simulink model "MGTestSystem_4bus"  (R2021b)
settings: Solver=VariableStepAuto  StartTime=0.0  StopTime=4  RelTol=1e-3
PreLoadFcn:
  | addpath Icons
  | addpath Util
InitFcn:
  | clc
  | %clear all
  | 
  | nDER = 4;
  | xssum = zeros(nDER*2,1);
  | save XSSUM xssum
  | 
  | Ts_Control=1e-4;       % local control time step
  | Ts_Simulation=5e-5;   %simulation time step
  | Ts_Power=5e-5;   % measurement time step
  | Tdisc=0.8;     % time setting for disconnecting from the main grid
  | 
  | Iref = 0.3;  % in p.u.
  | Iqref = 0;  % in p.u.
  | 
  | Ts_secondary =3e-2;   %  secondary control time step
  | %Ts_PMU = 1/60;
  | 
  | ft2km=3.0480e-04;
  | 
  | KPdroop=3.4e-4;
  | KQdroop=1e-3/1;
  | KPdroop2=4.5e-4;
  | KQdroop2=1.5e-3/1;
  | 
  | %KWinvdroop = 20.0;
  | %KVinvdroop = 16.7;
  | %KWinvdroop = 0.05;
  | %KVinvdroop = 0.08;
  | 
  | KWinvdroop = 1/(2*pi*KPdroop);
  | KVinvdroop = 1/(2*pi*KQdroop)
  | KWinvdroop2 = 1/(2*pi*KPdroop2);
  | KVinvdroop2 = 1/(2*pi*KQdroop2)
  | %KVinvdroop = 1/(KQdroop);
  | %KVinvdroop2 = 1/(KQdroop2);
  | %KWinvdroop = 1/(KPdroop);
  | %KWinvdroop2 = 1/(KPdroop2);
  | 
  | droopv1=1/KVinvdroop
  | droopv2=1/KVinvdroop2
  | 
  | 
  | 
  | 
  | wfilter = 35;
  | Rv=0.0;
  | Lv=0e-3;
  | 
  | div=1;
  | 
  | 
  | Kpac=0.1/1;
  | Kiac=420/1;
  | Kpaci=15/div;
  | Kiaci=2e3/div;
  | Kpac2=0.05/1;
  | Kiac2=390/1;
  | Kpaci2=15/div;
  | Kiaci2=1.6e3/div;
  | ... (+47 lines)
undefined symbols (not defined in the file or in its folder): D1, Delta, Ion, Lithium
libraries: spsStairGeneratorLib x24, spsThreePhaseSeriesRLCBranchLib x24, powerlib_extras x23, spsSeriesRLCBranchLib x20, spsThreePhaseVIMeasurementLib x18, slpidlib x18, spsThreePhaseBreakerLib x15, spsRMSLib x10, spsThreePhaseSeriesRLCLoadLib x8, spsVoltageMeasurementLib x8, spsPMUPLLBasedPositiveSequenceLib x6, spsPowerLib x5
(part 3 of 7)

== system MGTestSystem_4bus/Bus_6/PLL ==
  Vabc_LN_pu : Inport
  2pi60'1 : Constant  Value=2*pi*60
  2pi60'2 : Constant  Value=2*pi*60
  2pi60'3 : Constant  Value=2*pi*60
  Constant : Constant  Value=90
  Demux : Demux  Outputs=3
  Gain1 : Gain  Gain=180/pi  SaturateOnIntegerOverflow=on  OutDataTypeStr=Inherit: Same as input  ParamDataTypeStr=Inherit: Same as input
  Gain2 : Gain  Gain=180/pi  SaturateOnIntegerOverflow=on  OutDataTypeStr=Inherit: Same as input  ParamDataTypeStr=Inherit: Same as input
  Gain3 : Gain  Gain=180/pi  SaturateOnIntegerOverflow=on  OutDataTypeStr=Inherit: Same as input  ParamDataTypeStr=Inherit: Same as input
  Mux : Mux  Inputs=3
  Pll1 : Subsystem
  Pll2 : Subsystem
  Pll3 : Subsystem
  Sum : Sum  Inputs=|++
  delta_abc : Outport  VectorParamsAs1DForOutWhenUnconnected=off
  wires:
  Vabc_LN_pu/1 -> Demux/1
  Demux/1 -> Pll3/1(señal)
  2pi60'3/1 -> Pll3/2(w)
  Pll3/1(f cos (rad)) -> Gain1/1
  Demux/2 -> Pll1/1(señal)
  2pi60'1/1 -> Pll1/2(w)
  Gain2/1 -> Mux/2
  Demux/3 -> Pll2/1(señal)
  2pi60'2/1 -> Pll2/2(w)
  Pll2/1(f cos (rad)) -> Gain3/1
  Gain3/1 -> Mux/3
  Pll1/1(f cos (rad)) -> Gain2/1
  Mux/1 -> Sum/1
  Gain1/1 -> Mux/1
  Constant/1 -> Sum/2
  Sum/1 -> delta_abc/1

== system MGTestSystem_4bus/Bus_6/Power Factor Block1 ==
  Vabc : Inport
  Iabc : Inport  Port=2
  Complex to Magnitude-Angle : ComplexToMagnitudeAngle
  Mux : Mux  Inputs=2
  Mux1 : Mux  Inputs=2
  Power : spsPowerLib/Power  Freq=Freq  Vinit=Vinit  Iinit=Iinit  Ts=Ts
      settings: SourceProductBaseCode=PS
  RMS3 : spsRMSLib/RMS  TrueRMS=on  Freq=60  RMSInit=0  Ts=Ts_Simulation
  RMS4 : spsRMSLib/RMS  TrueRMS=on  Freq=60  RMSInit=0  Ts=Ts_Simulation
  Real-Imag to Complex : RealImagToComplex
  Terminator : Terminator
  compara : Gain  SaturateOnIntegerOverflow=on  OutDataTypeStr=Inherit: Same as input  ParamDataTypeStr=Inherit: Same as input
  cos(theta) : Trigonometry  Operator=cos
  to Kw : Gain  Gain=1/1000
  to Kw1 : Gain  Gain=1/1000
  Pabc : Outport  VectorParamsAs1DForOutWhenUnconnected=off
  Qabc : Outport  Port=2  VectorParamsAs1DForOutWhenUnconnected=off
  Vabc y Vabc (rms) : Outport  Port=3  VectorParamsAs1DForOutWhenUnconnected=off
  Iabc y Iabc (rms) : Outport  Port=4  VectorParamsAs1DForOutWhenUnconnected=off
  "PFabc " : Outport  Port=5  VectorParamsAs1DForOutWhenUnconnected=off
  tag scope: P_abc_Bus0=global, Q_abc_Bus0=global
  wires:
  Complex to Magnitude-Angle/2 -> cos(theta)/1
  Real-Imag to Complex/1 -> Complex to Magnitude-Angle/1
  cos(theta)/1 -> "PFabc "/1
  Complex to Magnitude-Angle/1 -> Terminator/1
  Iabc/1 -> RMS4/1, compara/1, Power/2
  RMS4/1 -> Mux1/2
  Mux1/1 -> Iabc y Iabc (rms)/1
  Mux/1 -> Vabc y Vabc (rms)/1
  Vabc/1 -> Power/1, Mux/2, RMS3/1
  compara/1 -> Mux1/1
  RMS3/1 -> Mux/1
  Power/1 -> to Kw1/1, Pabc/1, Real-Imag to Complex/1
  Power/2 -> Qabc/1, Real-Imag to Complex/2, to Kw/1
  to Kw/1 -> [Q_abc_Bus0]
  to Kw1/1 -> [P_abc_Bus0]

== system MGTestSystem_4bus/DATA  ADQUISITION/Delta_abc ==
  From10 : From  Commented=on  GotoTag=delta_abc_Bus8  TagVisibility=global
  From12 : From  Commented=on  GotoTag=delta_abc_Bus9  TagVisibility=global
  From13 : From  Commented=on  GotoTag=delta_abc_Bus10  TagVisibility=global
  From14 : From  Commented=on  GotoTag=delta_abc_Bus5  TagVisibility=global
  From15 : From  Commented=on  GotoTag=delta_abc_Bus11  TagVisibility=global
  From16 : From  Commented=on  GotoTag=delta_abc_Bus12  TagVisibility=global
  From17 : From  Commented=on  GotoTag=delta_abc_Bus13  TagVisibility=global
  From18 : From  Commented=on  GotoTag=delta_abc_Bus4L  TagVisibility=global
  From20 : From  Commented=on  GotoTag=delta_abc_Bus6  TagVisibility=global
  From22 : From  Commented=on  GotoTag=delta_abc_Bus4L  TagVisibility=global
  From23 : From  Commented=on  GotoTag=delta_abc_Bus7  TagVisibility=global
  From24 : From  Commented=on  GotoTag=delta_abc_Bus5L  TagVisibility=global
  From26 : From  Commented=on  GotoTag=delta_abc_Bus8  TagVisibility=global
  From29 : From  Commented=on  GotoTag=delta_abc_Bus9  TagVisibility=global
  From3 : From  Commented=on  GotoTag=delta_abc_Bus5  TagVisibility=global
  From32 : From  Commented=on  GotoTag=delta_abc_Bus10  TagVisibility=global
  From35 : From  Commented=on  GotoTag=delta_abc_Bus11  TagVisibility=global
  From38 : From  Commented=on  GotoTag=delta_abc_Bus12  TagVisibility=global
  From4 : From  Commented=on  GotoTag=delta_abc_Bus13  TagVisibility=global
  From41 : From  Commented=on  GotoTag=delta_abc_Bus4L  TagVisibility=global
  From7 : From  Commented=on  GotoTag=delta_abc_Bus6  TagVisibility=global
  From9 : From  Commented=on  GotoTag=delta_abc_Bus7  TagVisibility=global
  Mux3 : Mux  Inputs=15
  Scope : Scope  Commented=on  NumInputPorts=15
  f3 : ToWorkspace  Commented=on  VariableName=ang_abc  SaveFormat=Timeseries  SampleTime=-1
  wires:
  From32/1 -> Mux3/10
  [delta_abc_Bus4] -> Mux3/4
  From23/1 -> Mux3/7
  From26/1 -> Mux3/8
  From35/1 -> Mux3/11
  From14/1 -> Mux3/5
  From29/1 -> Mux3/9
  [delta_abc_Bus2] -> Mux3/2
  [delta_abc_Bus1] -> Mux3/1
  From38/1 -> Mux3/12
  From41/1 -> Mux3/14
  Mux3/1 -> f3/1
  From20/1 -> Mux3/6
  From17/1 -> Mux3/13
  [delta_abc_Bus3] -> Mux3/3
  [delta_abc_Bus3] -> Scope/3
  From4/1 -> Scope/13
  From7/1 -> Scope/6
  From13/1 -> Scope/10
  [delta_abc_Bus2] -> Scope/2
  [delta_abc_Bus1] -> Scope/1
  From3/1 -> Scope/5
  From16/1 -> Scope/12
  From15/1 -> Scope/11
  From10/1 -> Scope/8
  From18/1 -> Scope/14
  From12/1 -> Scope/9
  From9/1 -> Scope/7
  [delta_abc_Bus4] -> Scope/4
  From22/1 -> Scope/15
  From24/1 -> Mux3/15

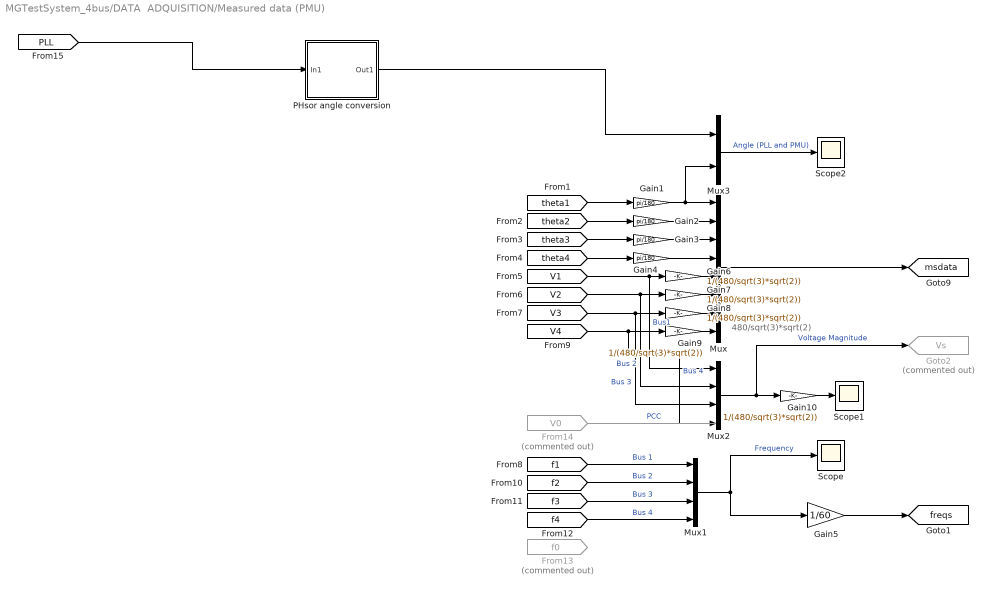
== system MGTestSystem_4bus/DATA  ADQUISITION/Measured data (PMU) ==
  note: 480/sqrt(3)*sqrt(2)
  From13 : From  Commented=on  GotoTag=f0  TagVisibility=global
  From14 : From  Commented=on  GotoTag=V0  TagVisibility=global
  Gain{1..4} (4 alike) : Gain  Gain=pi/180
  Gain{6..10} (5 alike) : Gain  Gain=1/(480/sqrt(3)*sqrt(2))
  Gain5 : Gain  Gain=1/60
  Goto2 : Goto  Commented=on  GotoTag=Vs  TagVisibility=global
  Mux : Mux  Inputs=8
  Mux1 : Mux
  Mux2 : Mux
  Mux3 : Mux  Inputs=2
  PHsor angle conversion : Subsystem
  Scope : Scope
  Scope1 : Scope
  Scope2 : Scope
  tag scope: freqs=global, msdata=global
  wires:
  [theta1] -> Gain1/1
  Mux/1 -> [msdata]
  [theta2] -> Gain2/1
  [V2] -> Mux2/2, Gain7/1  "Bus 2"
  [V3] -> Mux2/3, Gain8/1  "Bus 3"
  [V4] -> Mux2/4, Gain9/1  "Bus 4"
  [theta3] -> Gain3/1
  [theta4] -> Gain4/1
  [f1] -> Mux1/1  "Bus 1"
  [f2] -> Mux1/2  "Bus 2"
  [f3] -> Mux1/3  "Bus 3"
  [f4] -> Mux1/4  "Bus 4"
  Mux1/1 -> Scope/1, Gain5/1  "Frequency"
  [V1] -> Mux2/1, Gain6/1  "Bus1"
  Mux2/1 -> Goto2/1, Gain10/1  "Voltage Magnitude"
  Gain1/1 -> Mux3/2, Mux/1
  Gain2/1 -> Mux/2
  Gain3/1 -> Mux/3
  Gain4/1 -> Mux/4
  Gain5/1 -> [freqs]
  Gain6/1 -> Mux/5
  Gain7/1 -> Mux/6
  Gain8/1 -> Mux/7
  Gain9/1 -> Mux/8
  From14/1 -> ?  "PCC"
  Mux3/1 -> Scope2/1  "Angle (PLL and PMU)"
  [PLL] -> PHsor angle conversion/1(In1)
  PHsor angle conversion/1(Out1) -> Mux3/1
  Gain10/1 -> Scope1/1

== system MGTestSystem_4bus/DATA  ADQUISITION/PF_abc ==
  From11 : From  Commented=on  GotoTag=PFabc_Bus5  TagVisibility=global
  From17 : From  Commented=on  GotoTag=PFabc_Bus6  TagVisibility=global
  From20 : From  Commented=on  GotoTag=PFabc_Bus7  TagVisibility=global
  From23 : From  Commented=on  GotoTag=PFabc_Bus8  TagVisibility=global
  From26 : From  Commented=on  GotoTag=PFabc_Bus9  TagVisibility=global
  From29 : From  Commented=on  GotoTag=PFabc_Bus10  TagVisibility=global
  From32 : From  Commented=on  GotoTag=PFabc_Bus11  TagVisibility=global
  From35 : From  Commented=on  GotoTag=PFabc_Bus12  TagVisibility=global
  From38 : From  Commented=on  GotoTag=PFabc_Bus13  TagVisibility=global
  From41 : From  Commented=on  GotoTag=PFabc_Bus4L  TagVisibility=global
  Mux2 : Mux  Inputs=14
  f3 : ToWorkspace  Commented=on  VariableName=PF_abc  SaveFormat=Timeseries  SampleTime=-1
  wires:
  [PFabc_Bus2] -> Mux2/2
  [PFabc_Bus4] -> Mux2/4
  [PFabc_Bus1] -> Mux2/1
  From17/1 -> Mux2/6
  Mux2/1 -> f3/1
  From11/1 -> Mux2/5
  From41/1 -> Mux2/14
  From23/1 -> Mux2/8
  From26/1 -> Mux2/9
  From20/1 -> Mux2/7
  From32/1 -> Mux2/11
  From38/1 -> Mux2/13
  From29/1 -> Mux2/10
  [PFabc_Bus3] -> Mux2/3
  From35/1 -> Mux2/12

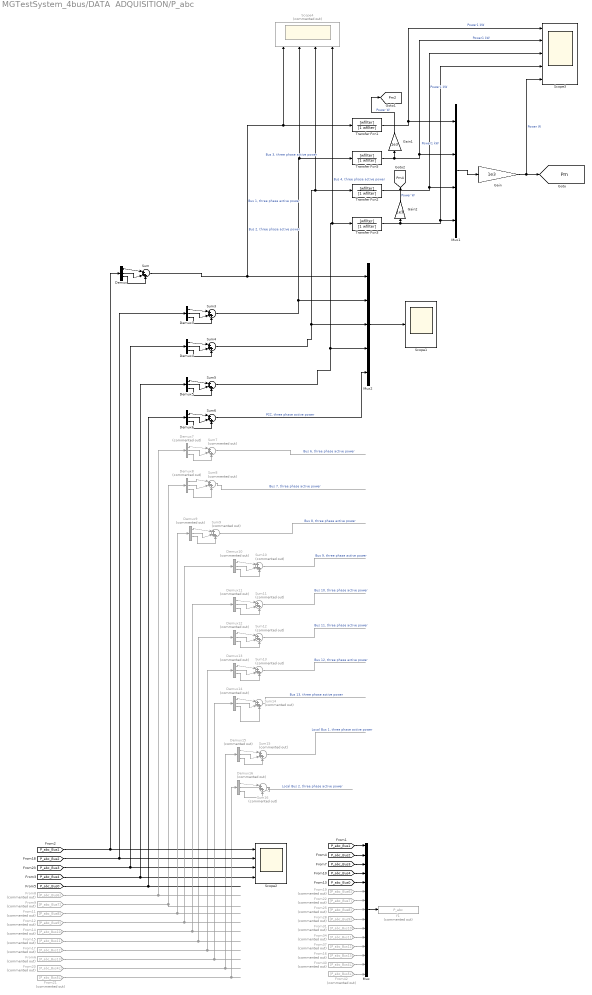
== system MGTestSystem_4bus/DATA  ADQUISITION/P_abc ==
  Demux{,3..6} (5 alike) : Demux  Outputs=3
  Demux{7..16} (10 alike) : Demux  Commented=on  Outputs=3
  From11 : From  Commented=on  GotoTag=P_abc_Bus8  TagVisibility=global
  From12 : From  Commented=on  GotoTag=P_abc_Bus9  TagVisibility=global
  From14 : From  Commented=on  GotoTag=P_abc_Bus10  TagVisibility=global
  From15 : From  Commented=on  GotoTag=P_abc_Bus11  TagVisibility=global
  From16 : From  Commented=on  GotoTag=P_abc_Bus13  TagVisibility=global
  From17 : From  Commented=on  GotoTag=P_abc_Bus12  TagVisibility=global
  From19 : From  Commented=on  GotoTag=P_abc_Bus6  TagVisibility=global
  From20 : From  Commented=on  GotoTag=P_abc_Bus4L  TagVisibility=global
  From21 : From  Commented=on  GotoTag=P_abc_Bus5L  TagVisibility=global
  From22 : From  Commented=on  GotoTag=P_abc_Bus7  TagVisibility=global
  From25 : From  Commented=on  GotoTag=P_abc_Bus8  TagVisibility=global
  From28 : From  Commented=on  GotoTag=P_abc_Bus9  TagVisibility=global
  From31 : From  Commented=on  GotoTag=P_abc_Bus10  TagVisibility=global
  From34 : From  Commented=on  GotoTag=P_abc_Bus11  TagVisibility=global
  From37 : From  Commented=on  GotoTag=P_abc_Bus12  TagVisibility=global
  From40 : From  Commented=on  GotoTag=P_abc_Bus4L  TagVisibility=global
  From42 : From  Commented=on  GotoTag=P_abc_Bus5L  TagVisibility=global
  From6 : From  Commented=on  GotoTag=P_abc_Bus13  TagVisibility=global
  From8 : From  Commented=on  GotoTag=P_abc_Bus6  TagVisibility=global
  From9 : From  Commented=on  GotoTag=P_abc_Bus7  TagVisibility=global
  Gain : Gain  Gain=1e3
  Gain1 : Gain  Gain=1e3
  Gain2 : Gain  Gain=1e3
  Mux : Mux  Inputs=15
  Mux1 : Mux
  Mux2 : Mux  Inputs=5
  Scope1 : Scope
  Scope2 : Scope  NumInputPorts=4
  Scope3 : Scope  NumInputPorts=5
  Scope4 : Scope  Commented=on  NumInputPorts=4
  Sum{,3..6} (5 alike) : Sum  Inputs=|+++
  Sum{7..16} (10 alike) : Sum  Commented=on  Inputs=|+++
  Transfer Fcn{1..3,5} (4 alike) : TransferFcn  Numerator=[wfilter]  Denominator=[1 wfilter]
  f1 : ToWorkspace  Commented=on  VariableName=P_abc  SaveFormat=Timeseries  SampleTime=-1
  tag scope: Pm2=global, Pm4=global, Pm=global
  wires:
  [P_abc_Bus1] -> Mux/1
  [P_abc_Bus3] -> Mux/3
  [P_abc_Bus2] -> Mux/2
  From16/1 -> Mux/13
  Mux/1 -> f1/1
  From37/1 -> Mux/12
  From28/1 -> Mux/9
  From25/1 -> Mux/8
  From31/1 -> Mux/10
  From34/1 -> Mux/11
  From22/1 -> Mux/7
  [P_abc_Bus4] -> Mux/4
  From40/1 -> Mux/14
  [P_abc_Bus0] -> Mux/5
  From42/1 -> Mux/15
  From19/1 -> Mux/6
  [P_abc_Bus4] -> Scope2/4, Demux5/1
  From17/1 -> Demux13/1
  From20/1 -> Demux15/1
  From15/1 -> Demux12/1
  From9/1 -> Demux8/1
  [P_abc_Bus3] -> Scope2/3, Demux4/1
  [P_abc_Bus2] -> Scope2/2, Demux3/1
  From6/1 -> Demux14/1
  From12/1 -> Demux10/1
  [P_abc_Bus0] -> Demux6/1
  From21/1 -> Demux16/1
  From8/1 -> Demux7/1
  [P_abc_Bus1] -> Scope2/1, Demux/1
  Demux/1 -> Sum/1
  Demux/2 -> Sum/2
  Demux/3 -> Sum/3
  Sum/1 -> Mux2/1, Transfer Fcn1/1, Scope4/1  "Bus 1, three phase active power"
  From11/1 -> Demux9/1
  From14/1 -> Demux11/1
  Demux3/3 -> Sum3/3
  Demux3/2 -> Sum3/2
  Sum3/1 -> Mux2/2, Transfer Fcn5/1, Scope4/2  "Bus 2, three phase active power"
  Demux3/1 -> Sum3/1
  Demux4/1 -> Sum4/1
  Sum4/1 -> Mux2/3, Transfer Fcn2/1, Scope4/3  "Bus 3, three phase active power"
  Demux4/2 -> Sum4/2
  Demux4/3 -> Sum4/3
  Demux5/3 -> Sum5/3
  Demux5/2 -> Sum5/2
  Sum5/1 -> Mux2/4, Transfer Fcn3/1, Scope4/4  "Bus 4, three phase active power"
  Demux5/1 -> Sum5/1
  Demux6/1 -> Sum6/1
  Sum6/1 -> Mux2/5  "PCC, three phase active power"
  Demux6/2 -> Sum6/2
  Demux6/3 -> Sum6/3
  Demux7/3 -> Sum7/3
  Demux7/2 -> Sum7/2
  Sum7/1 -> ?  "Bus 6, three phase active power"
  Demux7/1 -> Sum7/1
  Demux8/1 -> Sum8/1
  Sum8/1 -> ?  "Bus 7, three phase active power"
  Demux8/2 -> Sum8/2
  Demux8/3 -> Sum8/3
  Demux13/3 -> Sum13/3
  Sum13/1 -> ?  "Bus 12, three phase active power"
  Demux13/1 -> Sum13/1
  Demux13/2 -> Sum13/2
  Sum11/1 -> ?  "Bus 10, three phase active power"
  Demux11/1 -> Sum11/1
  Demux11/3 -> Sum11/3
  Demux11/2 -> Sum11/2
  Demux12/2 -> Sum12/2
  Sum12/1 -> ?  "Bus 11, three phase active power"
  Demux12/3 -> Sum12/3
  Demux12/1 -> Sum12/1
  Demux14/2 -> Sum14/2
  Sum14/1 -> ?  "Bus 13, three phase active power"
  Demux14/3 -> Sum14/3
  Demux14/1 -> Sum14/1
  Demux9/2 -> Sum9/2
  Demux9/1 -> Sum9/1
  Sum10/1 -> ?  "Bus 9, three phase active power"
  Demux10/1 -> Sum10/1
  Demux9/3 -> Sum9/3
  Demux10/2 -> Sum10/2
  Demux10/3 -> Sum10/3
  Sum9/1 -> ?  "Bus 8, three phase active power"
  Demux16/3 -> Sum16/3
  Demux15/2 -> Sum15/2
  Sum16/1 -> ?  "Local Bus 2, three phase active power"
  Demux15/1 -> Sum15/1
  Sum15/1 -> ?  "Local Bus 1, three phase active power"
  Demux15/3 -> Sum15/3
  Demux16/1 -> Sum16/1
  Demux16/2 -> Sum16/2
  Mux1/1 -> Gain/1
  Gain/1 -> Scope3/5, [Pm]  "Power W"
  Transfer Fcn1/1 -> Scope3/1, Mux1/1  "Power1 kW"
  Transfer Fcn5/1 -> Gain1/1, Scope3/2, Mux1/2  "Power1 kW"
  Transfer Fcn2/1 -> Scope3/3, Mux1/3  "Power1 kW"
  Transfer Fcn3/1 -> Scope3/4, Mux1/4, Gain2/1  "Power1 kW"
  Mux2/1 -> Scope1/1
  Gain1/1 -> [Pm2]  "Power W"
  Gain2/1 -> [Pm4]  "Power W"

== system MGTestSystem_4bus/DATA  ADQUISITION/Power_Losses_abc ==
  Mux : Mux  Inputs=14
  f2 : ToWorkspace  VariableName=Power_Losse_abc  SaveFormat=Timeseries  SampleTime=-1
  wires:
  [Power_Losse_abc_L12] -> Mux/12
  [Power_Losse_abc_L10] -> Mux/10
  [Power_Losse_abc_L13] -> Mux/13
  [Power_Losse_abc_L1] -> Mux/1
  Mux/1 -> f2/1
  [Power_Losse_abc_L2] -> Mux/2
  [Power_Losse_abc_L3] -> Mux/3
  [Power_Losse_abc_L4] -> Mux/4
  [Power_Losse_abc_L5] -> Mux/5
  [Power_Losse_abc_L14] -> Mux/14
  [Power_Losse_abc_L9] -> Mux/9
  [Power_Losse_abc_L6] -> Mux/6
  [Power_Losse_abc_L8] -> Mux/8
  [Power_Losse_abc_L11] -> Mux/11
  [Power_Losse_abc_L7] -> Mux/7

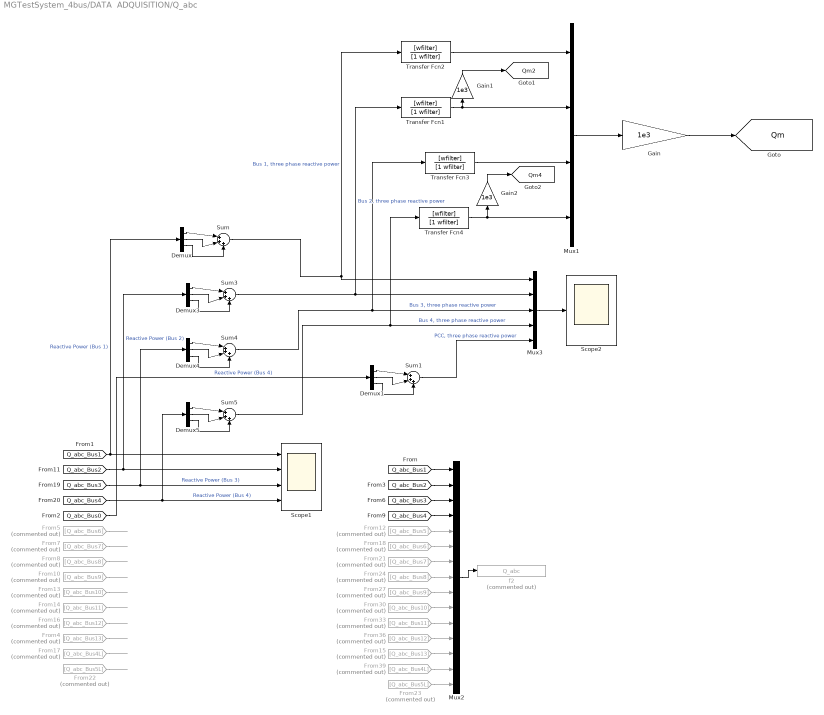
== system MGTestSystem_4bus/DATA  ADQUISITION/Q_abc ==
  Demux{,1,3..5} (5 alike) : Demux  Outputs=3
  From10 : From  Commented=on  GotoTag=Q_abc_Bus9  TagVisibility=global
  From12 : From  Commented=on  GotoTag=Q_abc_Bus5  TagVisibility=global
  From13 : From  Commented=on  GotoTag=Q_abc_Bus10  TagVisibility=global
  From14 : From  Commented=on  GotoTag=Q_abc_Bus11  TagVisibility=global
  From15 : From  Commented=on  GotoTag=Q_abc_Bus13  TagVisibility=global
  From16 : From  Commented=on  GotoTag=Q_abc_Bus12  TagVisibility=global
  From17 : From  Commented=on  GotoTag=Q_abc_Bus4L  TagVisibility=global
  From18 : From  Commented=on  GotoTag=Q_abc_Bus6  TagVisibility=global
  From21 : From  Commented=on  GotoTag=Q_abc_Bus7  TagVisibility=global
  From22 : From  Commented=on  GotoTag=Q_abc_Bus5L  TagVisibility=global
  From23 : From  Commented=on  GotoTag=Q_abc_Bus5L  TagVisibility=global
  From24 : From  Commented=on  GotoTag=Q_abc_Bus8  TagVisibility=global
  From27 : From  Commented=on  GotoTag=Q_abc_Bus9  TagVisibility=global
  From30 : From  Commented=on  GotoTag=Q_abc_Bus10  TagVisibility=global
  From33 : From  Commented=on  GotoTag=Q_abc_Bus11  TagVisibility=global
  From36 : From  Commented=on  GotoTag=Q_abc_Bus12  TagVisibility=global
  From39 : From  Commented=on  GotoTag=Q_abc_Bus4L  TagVisibility=global
  From4 : From  Commented=on  GotoTag=Q_abc_Bus13  TagVisibility=global
  From5 : From  Commented=on  GotoTag=Q_abc_Bus6  TagVisibility=global
  From7 : From  Commented=on  GotoTag=Q_abc_Bus7  TagVisibility=global
  From8 : From  Commented=on  GotoTag=Q_abc_Bus8  TagVisibility=global
  Gain : Gain  Gain=1e3
  Gain1 : Gain  Gain=1e3
  Gain2 : Gain  Gain=1e3
  Mux1 : Mux
  Mux2 : Mux  Inputs=15
  Mux3 : Mux  Inputs=5
  Scope1 : Scope  NumInputPorts=4
  Scope2 : Scope
  Sum{,1,3..5} (5 alike) : Sum  Inputs=|+++
  Transfer Fcn{1..4} (4 alike) : TransferFcn  Numerator=[wfilter]  Denominator=[1 wfilter]
  f2 : ToWorkspace  Commented=on  VariableName=Q_abc  SaveFormat=Timeseries  SampleTime=-1
  tag scope: Qm2=global, Qm4=global, Qm=global
  wires:
  Mux2/1 -> f2/1
  From18/1 -> Mux2/6
  [Q_abc_Bus1] -> Mux2/1
  [Q_abc_Bus4] -> Mux2/4
  From12/1 -> Mux2/5
  From27/1 -> Mux2/9
  From30/1 -> Mux2/10
  [Q_abc_Bus2] -> Mux2/2
  From36/1 -> Mux2/12
  From24/1 -> Mux2/8
  From15/1 -> Mux2/13
  [Q_abc_Bus3] -> Mux2/3
  From33/1 -> Mux2/11
  From39/1 -> Mux2/14
  From21/1 -> Mux2/7
  From7/1 -> ?
  From17/1 -> ?
  From14/1 -> ?
  [Q_abc_Bus3] -> Demux4/1, Scope1/3  "Reactive Power (Bus 3)"
  From4/1 -> ?
  From8/1 -> ?
  From16/1 -> ?
  [Q_abc_Bus2] -> Demux3/1, Scope1/2  "Reactive Power (Bus 2)"
  From13/1 -> ?
  From10/1 -> ?
  [Q_abc_Bus4] -> Demux5/1, Scope1/4  "Reactive Power (Bus 4)"
  [Q_abc_Bus1] -> Demux/1, Scope1/1  "Reactive Power (Bus 1)"
  From5/1 -> ?
  From22/1 -> ?
  From23/1 -> Mux2/15
  Demux3/2 -> Sum3/2
  Demux4/1 -> Sum4/1
  Demux3/3 -> Sum3/3
  Demux4/3 -> Sum4/3
  Demux5/2 -> Sum5/2
  Demux5/3 -> Sum5/3
  Demux5/1 -> Sum5/1
  Demux4/2 -> Sum4/2
  Demux3/1 -> Sum3/1
  Demux/1 -> Sum/1
  Demux/2 -> Sum/2
  Demux/3 -> Sum/3
  Sum/1 -> Transfer Fcn2/1, Mux3/1  "Bus 1, three phase reactive power"
  Sum3/1 -> Transfer Fcn1/1, Mux3/2  "Bus 2, three phase reactive power"
  Sum4/1 -> Transfer Fcn3/1, Mux3/3  "Bus 3, three phase reactive power"
  Sum5/1 -> Transfer Fcn4/1, Mux3/4  "Bus 4, three phase reactive power"
  Mux1/1 -> Gain/1
  Gain/1 -> [Qm]
  Transfer Fcn2/1 -> Mux1/1
  Transfer Fcn1/1 -> Mux1/2, Gain1/1
  Transfer Fcn3/1 -> Mux1/3
  Transfer Fcn4/1 -> Mux1/4, Gain2/1
  Mux3/1 -> Scope2/1
  Demux1/3 -> Sum1/3
  [Q_abc_Bus0] -> Demux1/1  "Reactive Power (Bus 4)"
  Demux1/2 -> Sum1/2
  Demux1/1 -> Sum1/1
  Sum1/1 -> Mux3/5  "PCC, three phase reactive power"
  Gain1/1 -> [Qm2]
  Gain2/1 -> [Qm4]

== system MGTestSystem_4bus/DATA  ADQUISITION/THDv_abc ==
  From12 : From  Commented=on  GotoTag=THDv_abc_Bus5  TagVisibility=global
  From18 : From  Commented=on  GotoTag=THDv_abc_Bus6  TagVisibility=global
  From21 : From  Commented=on  GotoTag=THDv_abc_Bus7  TagVisibility=global
  From24 : From  Commented=on  GotoTag=THDv_abc_Bus8  TagVisibility=global
  From27 : From  Commented=on  GotoTag=THDv_abc_Bus9  TagVisibility=global
  From30 : From  Commented=on  GotoTag=THDv_abc_Bus10  TagVisibility=global
  From33 : From  Commented=on  GotoTag=THDv_abc_Bus11  TagVisibility=global
  From36 : From  Commented=on  GotoTag=THDv_abc_Bus12  TagVisibility=global
  From39 : From  Commented=on  GotoTag=THDv_abc_Bus13  TagVisibility=global
  From42 : From  Commented=on  GotoTag=THDv_abc_Bus14
  Mux1 : Mux  Inputs=14
  f1 : ToWorkspace  Commented=on  VariableName=THDv_abc  SaveFormat=Timeseries  SampleTime=-1
  wires:
  From24/1 -> Mux1/8
  From12/1 -> Mux1/5
  [THDv_abc_Bus1] -> Mux1/1
  Mux1/1 -> f1/1
  From21/1 -> Mux1/7
  From33/1 -> Mux1/11
  [THDv_abc_Bus4] -> Mux1/4
  From27/1 -> Mux1/9
  From18/1 -> Mux1/6
  From42/1 -> Mux1/14
  [THDv_abc_Bus3] -> Mux1/3
  [THDv_abc_Bus2] -> Mux1/2
  From39/1 -> Mux1/13
  From30/1 -> Mux1/10
  From36/1 -> Mux1/12

== system MGTestSystem_4bus/DATA  ADQUISITION/VoltageLL_pu_abc ==
  From15 : From  Commented=on  GotoTag=Vabc_LL_Bus5  TagVisibility=global
  From16 : From  Commented=on  GotoTag=Vabc_LL_Bus6  TagVisibility=global
  From19 : From  Commented=on  GotoTag=Vabc_LL_Bus7  TagVisibility=global
  From2 : From  Commented=on  GotoTag=Vabc_LL_Bus5L  TagVisibility=global
  From22 : From  Commented=on  GotoTag=Vabc_LL_Bus8  TagVisibility=global
  From25 : From  Commented=on  GotoTag=Vabc_LL_Bus9  TagVisibility=global
  From28 : From  Commented=on  GotoTag=Vabc_LL_Bus10  TagVisibility=global
  From31 : From  Commented=on  GotoTag=Vabc_LL_Bus11  TagVisibility=global
  From34 : From  Commented=on  GotoTag=Vabc_LL_Bus12  TagVisibility=global
  From37 : From  Commented=on  GotoTag=Vabc_LL_Bus13  TagVisibility=global
  From40 : From  Commented=on  GotoTag=Vabc_LL_Bus4L  TagVisibility=global
  Mux : Mux  Inputs=15
  f2 : ToWorkspace  Commented=on  VariableName=VoltageLL_pu_abc  SaveFormat=Timeseries  SampleTime=-1
  wires:
  [Vabc_LL_Bus4] -> Mux/4
  [Vabc_LL_Bus3] -> Mux/3
  From15/1 -> Mux/5
  Mux/1 -> f2/1
  From22/1 -> Mux/8
  [Vabc_LL_Bus1] -> Mux/1
  [Vabc_LL_Bus2] -> Mux/2
  From31/1 -> Mux/11
  From34/1 -> Mux/12
  From16/1 -> Mux/6
  From40/1 -> Mux/14
  From19/1 -> Mux/7
  From2/1 -> Mux/15
  From37/1 -> Mux/13
  From25/1 -> Mux/9
  From28/1 -> Mux/10

== system MGTestSystem_4bus/DER 1/DC//DC 1 ==
  m_PV : Inport
  Boost Converter (Average Model) : Subsystem  mask(Boost Converter (Average Model)){Ts=Ts_Power}
      mask prompts: Ts "Sample time:"
      mask Display: disp('Boost\n(Average)')
  Bus Selector : BusSelector  OutputSignals=V_PV,I_PV
  Bus Selector1 : BusSelector  OutputSignals=V_PV,I_PV
  C : spsSeriesRLCBranchLib/Series RLC Branch  LConnTagsString=__new0  RConnTagsString=__new0  BranchType=C  Resistance=1.0  Inductance=1.0  SetiL0=off  InitialCurrent=0  Capacitance=100e-6  Setx0=on  InitialVoltage=260  Measurements=Branch voltage
  Constant : Constant
  Eliminate algebric loop2 : UnitDelay  InitialCondition=0.485  SampleTime=Ts_Control  HasFrameUpgradeWarning=on
  L1 : spsSeriesRLCBranchLib/Series RLC Branch  LConnTagsString=__new0  RConnTagsString=__new0  BranchType=RL  Resistance=0.005  Inductance=5e-3  SetiL0=off  InitialCurrent=0  Capacitance=1e-6  Setx0=off  InitialVoltage=0  Measurements=None
  MPPT Parameters : Subsystem
  "MPPT Control  " : MATLAB Function  TreatAsAtomicUnit=on
  Mean : spsMeanLib/Mean  Freq=60  Vinit=100  Ts=Ts_Control
  Product : Product  RndMeth=Zero
  WkW : Gain  Gain=1/1000
  " +" : PMIOPort  Side=Right
  +PV : PMIOPort  Port=2  Side=Left
  -PV : PMIOPort  Port=3  Side=Left
  " -" : PMIOPort  Port=4  Side=Right
  wires:
  "MPPT Control  "/1(D) -> Eliminate algebric loop2/1
  MPPT Parameters/1(Param) -> "MPPT Control  "/1(Param)
  Eliminate algebric loop2/1 -> Boost Converter (Average Model)/1(D)
  m_PV/1 -> Bus Selector1/1, Bus Selector/1
  Bus Selector/1 -> "MPPT Control  "/3(V)  "<V_PV>"
  Bus Selector/2 -> "MPPT Control  "/4(I)  "<I_PV>"
  Bus Selector1/1 -> Product/1  "<V_PV>"
  Product/1 -> WkW/1
  Bus Selector1/2 -> Product/2  "<I_PV>"
  WkW/1 -> Mean/1  "Pmean_PV (kW)"
  Mean/1 -> ?
  Constant/1 -> "MPPT Control  "/2(Enabled)
  connections:
  C/LConn1 -- +PV/RConn1 -- L1/LConn1
  L1/RConn1 -- Boost Converter (Average Model)/LConn1
  C/RConn1 -- Boost Converter (Average Model)/RConn2 -- " -"/RConn1 -- -PV/RConn1
  Boost Converter (Average Model)/RConn1 -- " +"/RConn1

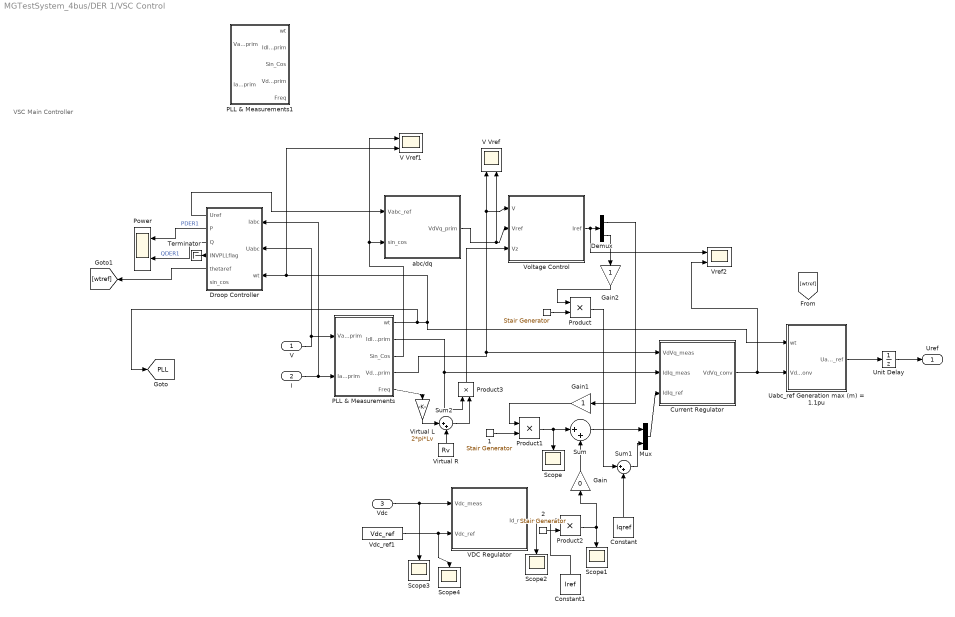
== system MGTestSystem_4bus/DER 1/VSC Control ==
  note: VSC Main Controller
  V : Inport  PortDimensions=3
  I : Inport  Port=2  PortDimensions=3
  Vdc : Inport  Port=3  PortDimensions=1
  " " : spsStairGeneratorLib/Stair Generator  t=[0,Tdisc]  e=[1,1]  Ts=Ts_Simulation
  " 1" : spsStairGeneratorLib/Stair Generator  t=[0,Tdisc]  e=[1,1]  Ts=Ts_Simulation
  " 2" : spsStairGeneratorLib/Stair Generator  t=[Ts_Simulation Tdisc]  e=[1 0]  Ts=Ts_Simulation
  Constant : Constant  Value=Iqref
  Constant1 : Constant  Value=Iref
  Current Regulator : Subsystem
  Demux : Demux  Outputs=2
  Droop Controller : Subsystem
  Gain : Gain  Gain=0
  Gain1 : Gain
  Gain2 : Gain
  Mux : Mux  Inputs=2
  PLL & Measurements : Subsystem
  PLL & Measurements1 : Subsystem
  Power : Scope  NumInputPorts=2
  Product{,1..3} (4 alike) : Product
  Scope{,1..4} (5 alike) : Scope
  Sum : Sum  Inputs=|++
  Sum1 : Sum  Inputs=|++
  Sum2 : Sum  Inputs=|++
  Terminator : Terminator
  Uabc_ref Generation max (m) = 1.1pu : Subsystem
  Unit Delay : UnitDelay  SampleTime=Ts_Control  HasFrameUpgradeWarning=on
  V Vref : Scope  NumInputPorts=2
  V Vref1 : Scope  NumInputPorts=2
  VDC Regulator : Subsystem
  Vdc_ref1 : Constant  Value=Vdc_ref
  Virtual L : Gain  Gain=2*pi*Lv
  Virtual R : Constant  Value=Rv
  Voltage Control : Subsystem
  Vref2 : Scope  NumInputPorts=2
  abc/dq : Subsystem
  Uref : Outport  VectorParamsAs1DForOutWhenUnconnected=off
  tag scope: PLL=global
  wires:
  Virtual L/1 -> Sum2/1
  Virtual R/1 -> Sum2/2
  Sum2/1 -> Product3/2
  PLL & Measurements/5(Freq) -> Virtual L/1
  Product3/1 -> Voltage Control/3(Vz)
  Product2/1 -> Scope1/1, Gain/1
  VDC Regulator/1(Id_ref) -> Scope2/1
  " 2"/1 -> Product2/2
  Product1/1 -> Sum/1, Scope/1
  Gain1/1 -> Product1/1
  " 1"/1 -> Product1/2
  Product/1 -> Sum1/1
  Gain2/1 -> Product/1
  " "/1 -> Product/2
  Sum1/1 -> Mux/2
  Constant/1 -> Sum1/2
  Gain/1 -> Sum/2
  Sum/1 -> Mux/1
  Mux/1 -> Current Regulator/3(IdIq_ref)
  Demux/2 -> Gain2/1
  Demux/1 -> Gain1/1
  Voltage Control/1(Iref) -> Vref2/1, Demux/1
  Droop Controller/4(INVPLLflag) -> Terminator/1
  PLL & Measurements/3(Sin_Cos) -> abc/dq/2(sin_cos), V Vref1/1
  PLL & Measurements/4(VdVq_prim) -> V Vref/1, Voltage Control/1(V), Current Regulator/1(VdVq_meas)
  abc/dq/1(VdVq_prim) -> V Vref/2, Voltage Control/2(Vref)
  Droop Controller/1(Uref) -> abc/dq/1(Vabc_ref)
  Droop Controller/3(Q) -> Power/2  "QDER1"
  Droop Controller/2(P) -> Power/1  "PDER1"
  Vdc_ref1/1 -> VDC Regulator/2(Vdc_ref), Scope4/1
  Uabc_ref Generation max (m) = 1.1pu/1(Uabc_ref) -> Unit Delay/1
  Unit Delay/1 -> Uref/1
  I/1 -> PLL & Measurements/2(Iabc_prim), Droop Controller/1(Iabc)
  V/1 -> PLL & Measurements/1(Vabc_prim), Droop Controller/2(Uabc)
  Vdc/1 -> Scope3/1, VDC Regulator/1(Vdc_meas)
  PLL & Measurements/2(IdIq_prim) -> Product3/1, Current Regulator/2(IdIq_meas)
  Current Regulator/1(VdVq_conv) -> Vref2/2, Uabc_ref Generation max (m) = 1.1pu/2(VdVq_conv)
  PLL & Measurements/1(wt) -> [PLL], Uabc_ref Generation max (m) = 1.1pu/1(wt), Droop Controller/3(wt), V Vref1/2
  Constant1/1 -> Product2/1
  Droop Controller/5(thetaref) -> [wtref]

== system MGTestSystem_4bus/DER 2/DC//DC 1 ==
  m_PV : Inport
  Boost Converter (Average Model) : Subsystem  mask(Boost Converter (Average Model)){Ts=Ts_Power}
      mask prompts: Ts "Sample time:"
      mask Display: disp('Boost\n(Average)')
  Bus Selector : BusSelector  OutputSignals=V_PV,I_PV
  Bus Selector1 : BusSelector  OutputSignals=V_PV,I_PV
  C : spsSeriesRLCBranchLib/Series RLC Branch  LConnTagsString=__new0  RConnTagsString=__new0  BranchType=C  Resistance=1.0  Inductance=1.0  SetiL0=off  InitialCurrent=0  Capacitance=100e-6  Setx0=on  InitialVoltage=260  Measurements=Branch voltage
  Constant : Constant
  Eliminate algebric loop2 : UnitDelay  InitialCondition=0.485  SampleTime=Ts_Control  HasFrameUpgradeWarning=on
  L1 : spsSeriesRLCBranchLib/Series RLC Branch  LConnTagsString=__new0  RConnTagsString=__new0  BranchType=RL  Resistance=0.005  Inductance=5e-3  SetiL0=off  InitialCurrent=0  Capacitance=1e-6  Setx0=off  InitialVoltage=0  Measurements=None
  MPPT Parameters : Subsystem
  "MPPT Control  " : MATLAB Function  TreatAsAtomicUnit=on
  Mean : spsMeanLib/Mean  Freq=60  Vinit=100  Ts=Ts_Control
  Product : Product  RndMeth=Zero
  WkW : Gain  Gain=1/1000
  " +" : PMIOPort  Side=Right
  +PV : PMIOPort  Port=2  Side=Left
  -PV : PMIOPort  Port=3  Side=Left
  " -" : PMIOPort  Port=4  Side=Right
  wires:
  "MPPT Control  "/1(D) -> Eliminate algebric loop2/1
  MPPT Parameters/1(Param) -> "MPPT Control  "/1(Param)
  Eliminate algebric loop2/1 -> Boost Converter (Average Model)/1(D)
  m_PV/1 -> Bus Selector1/1, Bus Selector/1
  Bus Selector/1 -> "MPPT Control  "/3(V)  "<V_PV>"
  Bus Selector/2 -> "MPPT Control  "/4(I)  "<I_PV>"
  Bus Selector1/1 -> Product/1  "<V_PV>"
  Product/1 -> WkW/1
  Bus Selector1/2 -> Product/2  "<I_PV>"
  WkW/1 -> Mean/1  "Pmean_PV (kW)"
  Mean/1 -> ?
  Constant/1 -> "MPPT Control  "/2(Enabled)
  connections:
  C/LConn1 -- +PV/RConn1 -- L1/LConn1
  L1/RConn1 -- Boost Converter (Average Model)/LConn1
  C/RConn1 -- Boost Converter (Average Model)/RConn2 -- " -"/RConn1 -- -PV/RConn1
  Boost Converter (Average Model)/RConn1 -- " +"/RConn1

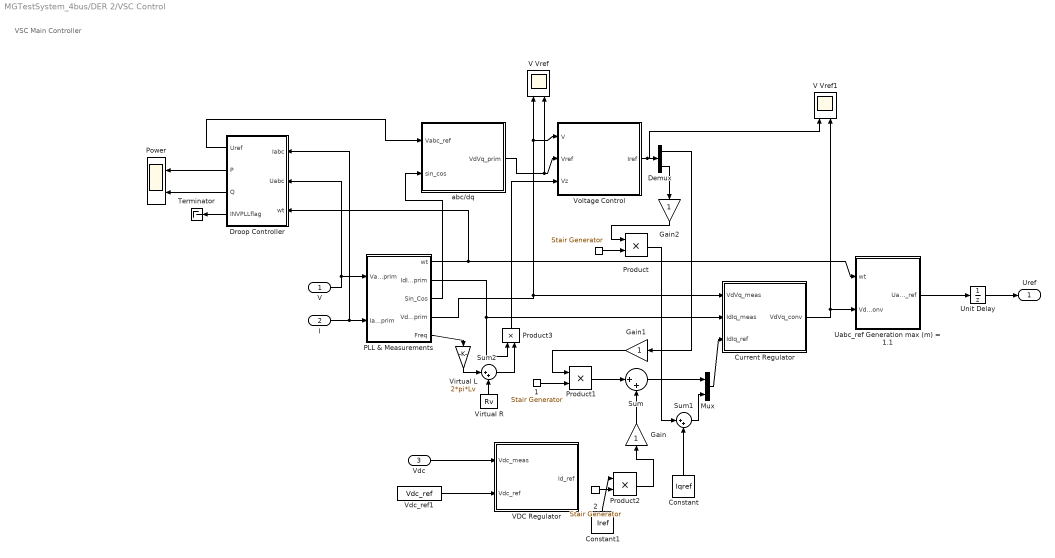
== system MGTestSystem_4bus/DER 2/VSC Control ==
  note: VSC Main Controller
  V : Inport  PortDimensions=3
  I : Inport  Port=2  PortDimensions=3
  Vdc : Inport  Port=3  PortDimensions=1
  " " : spsStairGeneratorLib/Stair Generator  t=[Tdisc]  e=[1]  Ts=Ts_Simulation
  " 1" : spsStairGeneratorLib/Stair Generator  t=[Tdisc]  e=[1]  Ts=Ts_Simulation
  " 2" : spsStairGeneratorLib/Stair Generator  t=[Ts_Simulation Tdisc]  e=[1 0]  Ts=Ts_Simulation
  Constant : Constant  Value=Iqref
  Constant1 : Constant  Value=Iref
  Current Regulator : Subsystem
  Demux : Demux  Outputs=2
  Droop Controller : Subsystem
  Gain : Gain
  Gain1 : Gain
  Gain2 : Gain
  Mux : Mux  Inputs=2
  PLL & Measurements : Subsystem
  Power : Scope  NumInputPorts=2
  Product{,1..3} (4 alike) : Product
  Sum : Sum  Inputs=|++
  Sum1 : Sum  Inputs=|++
  Sum2 : Sum  Inputs=|++
  Terminator : Terminator
  Uabc_ref Generation max (m) = 1.1 : Subsystem
  Unit Delay : UnitDelay  SampleTime=Ts_Control  HasFrameUpgradeWarning=on
  V Vref : Scope  NumInputPorts=2
  V Vref1 : Scope  NumInputPorts=2
  VDC Regulator : Subsystem
  Vdc_ref1 : Constant  Value=Vdc_ref
  Virtual L : Gain  Gain=2*pi*Lv
  Virtual R : Constant  Value=Rv
  Voltage Control : Subsystem
  abc/dq : Subsystem
  Uref : Outport  VectorParamsAs1DForOutWhenUnconnected=off
  wires:
  Virtual L/1 -> Sum2/1
  Virtual R/1 -> Sum2/2
  Sum2/1 -> Product3/2
  PLL & Measurements/5(Freq) -> Virtual L/1
  Product3/1 -> Voltage Control/3(Vz)
  Product2/1 -> Gain/1
  " 2"/1 -> Product2/2
  Product1/1 -> Sum/1
  Gain1/1 -> Product1/1
  " 1"/1 -> Product1/2
  Product/1 -> Sum1/1
  Gain2/1 -> Product/1
  " "/1 -> Product/2
  Sum1/1 -> Mux/2
  Constant/1 -> Sum1/2
  Gain/1 -> Sum/2
  Sum/1 -> Mux/1
  Mux/1 -> Current Regulator/3(IdIq_ref)
  Demux/2 -> Gain2/1
  Demux/1 -> Gain1/1
  Voltage Control/1(Iref) -> V Vref1/1, Demux/1
  Droop Controller/4(INVPLLflag) -> Terminator/1
  PLL & Measurements/3(Sin_Cos) -> abc/dq/2(sin_cos)
  PLL & Measurements/4(VdVq_prim) -> V Vref/1, Voltage Control/1(V), Current Regulator/1(VdVq_meas)
  abc/dq/1(VdVq_prim) -> V Vref/2, Voltage Control/2(Vref)
  Droop Controller/1(Uref) -> abc/dq/1(Vabc_ref)
  Droop Controller/3(Q) -> Power/2
  Droop Controller/2(P) -> Power/1
  Vdc_ref1/1 -> VDC Regulator/2(Vdc_ref)
  Uabc_ref Generation max (m) = 1.1/1(Uabc_ref) -> Unit Delay/1
  Unit Delay/1 -> Uref/1
  I/1 -> PLL & Measurements/2(Iabc_prim), Droop Controller/1(Iabc)
  V/1 -> PLL & Measurements/1(Vabc_prim), Droop Controller/2(Uabc)
  Vdc/1 -> VDC Regulator/1(Vdc_meas)
  PLL & Measurements/2(IdIq_prim) -> Product3/1, Current Regulator/2(IdIq_meas)
  Current Regulator/1(VdVq_conv) -> Uabc_ref Generation max (m) = 1.1/2(VdVq_conv), V Vref1/2
  PLL & Measurements/1(wt) -> Droop Controller/3(wt), Uabc_ref Generation max (m) = 1.1/1(wt)
  Constant1/1 -> Product2/1

== system MGTestSystem_4bus/DER 3/DC//DC 1 ==
  m_PV : Inport
  Boost Converter (Average Model) : Subsystem  mask(Boost Converter (Average Model)){Ts=Ts_Power}
      mask prompts: Ts "Sample time:"
      mask Display: disp('Boost\n(Average)')
  Bus Selector : BusSelector  OutputSignals=V_PV,I_PV
  Bus Selector1 : BusSelector  OutputSignals=V_PV,I_PV
  C : spsSeriesRLCBranchLib/Series RLC Branch  LConnTagsString=__new0  RConnTagsString=__new0  BranchType=C  Resistance=1.0  Inductance=1.0  SetiL0=off  InitialCurrent=0  Capacitance=100e-6  Setx0=on  InitialVoltage=260  Measurements=Branch voltage
  Constant : Constant
  Eliminate algebric loop2 : UnitDelay  InitialCondition=0.485  SampleTime=Ts_Control  HasFrameUpgradeWarning=on
  L1 : spsSeriesRLCBranchLib/Series RLC Branch  LConnTagsString=__new0  RConnTagsString=__new0  BranchType=RL  Resistance=0.005  Inductance=5e-3  SetiL0=off  InitialCurrent=0  Capacitance=1e-6  Setx0=off  InitialVoltage=0  Measurements=None
  MPPT Parameters : Subsystem
  "MPPT Control  " : MATLAB Function  TreatAsAtomicUnit=on
  Mean : spsMeanLib/Mean  Freq=60  Vinit=100  Ts=Ts_Control
  Product : Product  RndMeth=Zero
  WkW : Gain  Gain=1/1000
  " +" : PMIOPort  Side=Right
  +PV : PMIOPort  Port=2  Side=Left
  -PV : PMIOPort  Port=3  Side=Left
  " -" : PMIOPort  Port=4  Side=Right
  wires:
  "MPPT Control  "/1(D) -> Eliminate algebric loop2/1
  MPPT Parameters/1(Param) -> "MPPT Control  "/1(Param)
  Eliminate algebric loop2/1 -> Boost Converter (Average Model)/1(D)
  m_PV/1 -> Bus Selector1/1, Bus Selector/1
  Bus Selector/1 -> "MPPT Control  "/3(V)  "<V_PV>"
  Bus Selector/2 -> "MPPT Control  "/4(I)  "<I_PV>"
  Bus Selector1/1 -> Product/1  "<V_PV>"
  Product/1 -> WkW/1
  Bus Selector1/2 -> Product/2  "<I_PV>"
  WkW/1 -> Mean/1  "Pmean_PV (kW)"
  Constant/1 -> "MPPT Control  "/2(Enabled)
  connections:
  C/LConn1 -- +PV/RConn1 -- L1/LConn1
  L1/RConn1 -- Boost Converter (Average Model)/LConn1
  C/RConn1 -- Boost Converter (Average Model)/RConn2 -- " -"/RConn1 -- -PV/RConn1
  Boost Converter (Average Model)/RConn1 -- " +"/RConn1

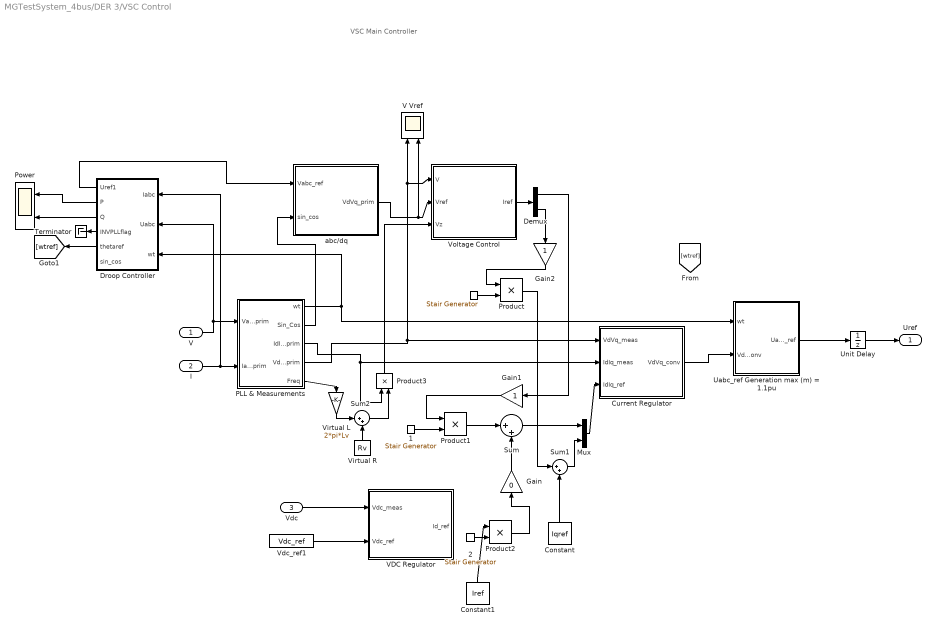
== system MGTestSystem_4bus/DER 3/VSC Control ==
  note: VSC Main Controller
  V : Inport  PortDimensions=3
  I : Inport  Port=2  PortDimensions=3
  Vdc : Inport  Port=3  PortDimensions=1
  " " : spsStairGeneratorLib/Stair Generator  t=[0,Tdisc]  e=[1,1]  Ts=Ts_Simulation
  " 1" : spsStairGeneratorLib/Stair Generator  t=[0,Tdisc]  e=[1,1]  Ts=Ts_Simulation
  " 2" : spsStairGeneratorLib/Stair Generator  t=[0 Tdisc]  e=[1 0]  Ts=Ts_Simulation
  Constant : Constant  Value=Iqref
  Constant1 : Constant  Value=Iref
  Current Regulator : Subsystem
  Demux : Demux  Outputs=2
  Droop Controller : Subsystem
  Gain : Gain  Gain=0
  Gain1 : Gain
  Gain2 : Gain
  Mux : Mux  Inputs=2
  PLL & Measurements : Subsystem
  Power : Scope  NumInputPorts=2
  Product{,1..3} (4 alike) : Product
  Sum : Sum  Inputs=|++
  Sum1 : Sum  Inputs=|++
  Sum2 : Sum  Inputs=|++
  Terminator : Terminator
  Uabc_ref Generation max (m) = 1.1pu : Subsystem
  Unit Delay : UnitDelay  SampleTime=Ts_Control  HasFrameUpgradeWarning=on
  V Vref : Scope  NumInputPorts=2
  VDC Regulator : Subsystem
  Vdc_ref1 : Constant  Value=Vdc_ref
  Virtual L : Gain  Gain=2*pi*Lv
  Virtual R : Constant  Value=Rv
  Voltage Control : Subsystem
  abc/dq : Subsystem
  Uref : Outport  VectorParamsAs1DForOutWhenUnconnected=off
  wires:
  Virtual L/1 -> Sum2/1
  Virtual R/1 -> Sum2/2
  Sum2/1 -> Product3/2
  PLL & Measurements/5(Freq) -> Virtual L/1
  Product3/1 -> Voltage Control/3(Vz)
  Product2/1 -> Gain/1
  " 2"/1 -> Product2/2
  Product1/1 -> Sum/1
  Gain1/1 -> Product1/1
  " 1"/1 -> Product1/2
  Product/1 -> Sum1/1
  Gain2/1 -> Product/1
  " "/1 -> Product/2
  Sum1/1 -> Mux/2
  Constant/1 -> Sum1/2
  Gain/1 -> Sum/2
  Sum/1 -> Mux/1
  Mux/1 -> Current Regulator/3(IdIq_ref)
  Demux/2 -> Gain2/1
  Demux/1 -> Gain1/1
  Voltage Control/1(Iref) -> Demux/1
  Droop Controller/4(INVPLLflag) -> Terminator/1
  PLL & Measurements/4(VdVq_prim) -> V Vref/1, Voltage Control/1(V), Current Regulator/1(VdVq_meas)
  abc/dq/1(VdVq_prim) -> V Vref/2, Voltage Control/2(Vref)
  Droop Controller/1(Uref1) -> abc/dq/1(Vabc_ref)
  Droop Controller/3(Q) -> Power/2
  Droop Controller/2(P) -> Power/1
  Vdc_ref1/1 -> VDC Regulator/2(Vdc_ref)
  Uabc_ref Generation max (m) = 1.1pu/1(Uabc_ref) -> Unit Delay/1
  Unit Delay/1 -> Uref/1
  I/1 -> PLL & Measurements/2(Iabc_prim), Droop Controller/1(Iabc)
  V/1 -> PLL & Measurements/1(Vabc_prim), Droop Controller/2(Uabc)
  Vdc/1 -> VDC Regulator/1(Vdc_meas)
  PLL & Measurements/3(IdIq_prim) -> Product3/1, Current Regulator/2(IdIq_meas)
  Current Regulator/1(VdVq_conv) -> Uabc_ref Generation max (m) = 1.1pu/2(VdVq_conv)
  PLL & Measurements/1(wt) -> Droop Controller/3(wt), Uabc_ref Generation max (m) = 1.1pu/1(wt)
  Constant1/1 -> Product2/1
  Droop Controller/5(thetaref) -> [wtref]
  PLL & Measurements/2(Sin_Cos) -> abc/dq/2(sin_cos)

== system MGTestSystem_4bus/DER 4/DC//DC 1 ==
  m_PV : Inport
  Boost Converter (Average Model) : Subsystem  mask(Boost Converter (Average Model)){Ts=Ts_Power}
      mask prompts: Ts "Sample time:"
      mask Display: disp('Boost\n(Average)')
  Bus Selector : BusSelector  OutputSignals=V_PV,I_PV
  Bus Selector1 : BusSelector  OutputSignals=V_PV,I_PV
  C : spsSeriesRLCBranchLib/Series RLC Branch  LConnTagsString=__new0  RConnTagsString=__new0  BranchType=C  Resistance=1.0  Inductance=1.0  SetiL0=off  InitialCurrent=0  Capacitance=100e-6  Setx0=on  InitialVoltage=260  Measurements=Branch voltage
  Constant : Constant
  Eliminate algebric loop2 : UnitDelay  InitialCondition=0.485  SampleTime=Ts_Control  HasFrameUpgradeWarning=on
  L1 : spsSeriesRLCBranchLib/Series RLC Branch  LConnTagsString=__new0  RConnTagsString=__new0  BranchType=RL  Resistance=0.005  Inductance=5e-3  SetiL0=off  InitialCurrent=0  Capacitance=1e-6  Setx0=off  InitialVoltage=0  Measurements=None
  MPPT Parameters : Subsystem
  "MPPT Control  " : MATLAB Function  TreatAsAtomicUnit=on
  Mean : spsMeanLib/Mean  Freq=60  Vinit=100  Ts=Ts_Control
  Product : Product  RndMeth=Zero
  WkW : Gain  Gain=1/1000
  " +" : PMIOPort  Side=Right
  +PV : PMIOPort  Port=2  Side=Left
  -PV : PMIOPort  Port=3  Side=Left
  " -" : PMIOPort  Port=4  Side=Right
  wires:
  "MPPT Control  "/1(D) -> Eliminate algebric loop2/1
  MPPT Parameters/1(Param) -> "MPPT Control  "/1(Param)
  Eliminate algebric loop2/1 -> Boost Converter (Average Model)/1(D)
  m_PV/1 -> Bus Selector1/1, Bus Selector/1
  Bus Selector/1 -> "MPPT Control  "/3(V)  "<V_PV>"
  Bus Selector/2 -> "MPPT Control  "/4(I)  "<I_PV>"
  Bus Selector1/1 -> Product/1  "<V_PV>"
  Product/1 -> WkW/1
  Bus Selector1/2 -> Product/2  "<I_PV>"
  WkW/1 -> Mean/1  "Pmean_PV (kW)"
  Mean/1 -> ?
  Constant/1 -> "MPPT Control  "/2(Enabled)
  connections:
  C/LConn1 -- +PV/RConn1 -- L1/LConn1
  L1/RConn1 -- Boost Converter (Average Model)/LConn1
  C/RConn1 -- Boost Converter (Average Model)/RConn2 -- " -"/RConn1 -- -PV/RConn1
  Boost Converter (Average Model)/RConn1 -- " +"/RConn1

== system MGTestSystem_4bus/DER 4/VSC Control ==
  note: VSC Main Controller
  V : Inport  PortDimensions=3
  I : Inport  Port=2  PortDimensions=3
  Vdc : Inport  Port=3  PortDimensions=1
  " " : spsStairGeneratorLib/Stair Generator  t=[Tdisc]  e=[1]  Ts=Ts_Simulation
  " 1" : spsStairGeneratorLib/Stair Generator  t=[Tdisc]  e=[1]  Ts=Ts_Simulation
  " 2" : spsStairGeneratorLib/Stair Generator  t=[Ts_Simulation Tdisc]  e=[1 0]  Ts=Ts_Simulation
  Constant : Constant  Value=Iqref
  Constant1 : Constant  Value=Iref
  Current Regulator : Subsystem
  Demux : Demux  Outputs=2
  Droop Controller : Subsystem
  Gain : Gain
  Gain1 : Gain
  Gain2 : Gain
  Mux : Mux  Inputs=2
  PLL & Measurements : Subsystem
  Power : Scope  NumInputPorts=2
  Product{,1..3} (4 alike) : Product
  Sum : Sum  Inputs=|++
  Sum1 : Sum  Inputs=|++
  Sum2 : Sum  Inputs=|++
  Terminator : Terminator
  Uabc_ref Generation max (m) = 1.1 : Subsystem
  Unit Delay : UnitDelay  SampleTime=Ts_Control  HasFrameUpgradeWarning=on
  V Vref : Scope  NumInputPorts=2
  VDC Regulator : Subsystem
  Vdc_ref1 : Constant  Value=Vdc_ref
  Virtual L : Gain  Gain=2*pi*Lv
  Virtual R : Constant  Value=Rv
  Voltage Control : Subsystem
  Vref2 : Scope  NumInputPorts=2
  abc/dq : Subsystem
  Uref : Outport  VectorParamsAs1DForOutWhenUnconnected=off
  wires:
  PLL & Measurements/1(wt) -> Uabc_ref Generation max (m) = 1.1/1(wt), Droop Controller/3(wt)
  Current Regulator/1(VdVq_conv) -> Vref2/2, Uabc_ref Generation max (m) = 1.1/2(VdVq_conv)
  PLL & Measurements/2(IdIq_prim) -> Current Regulator/2(IdIq_meas), Product3/1
  Vdc/1 -> VDC Regulator/1(Vdc_meas)
  V/1 -> Droop Controller/2(Uabc), PLL & Measurements/1(Vabc_prim)
  I/1 -> Droop Controller/1(Iabc), PLL & Measurements/2(Iabc_prim)
  Unit Delay/1 -> Uref/1
  Uabc_ref Generation max (m) = 1.1/1(Uabc_ref) -> Unit Delay/1
  Vdc_ref1/1 -> VDC Regulator/2(Vdc_ref)
  Droop Controller/2(P) -> Power/1
  Droop Controller/3(Q) -> Power/2
  Droop Controller/1(Uref) -> abc/dq/1(Vabc_ref)
  abc/dq/1(VdVq_prim) -> Voltage Control/2(Vref), V Vref/2
  PLL & Measurements/4(VdVq_prim) -> Current Regulator/1(VdVq_meas), Voltage Control/1(V), V Vref/1
  PLL & Measurements/3(Sin_Cos) -> abc/dq/2(sin_cos)
  Droop Controller/4(INVPLLflag) -> Terminator/1
  Voltage Control/1(Iref) -> Vref2/1, Demux/1
  Demux/1 -> Gain1/1
  Demux/2 -> Gain2/1
  Mux/1 -> Current Regulator/3(IdIq_ref)
  Sum/1 -> Mux/1
  Gain/1 -> Sum/2
  Constant/1 -> Sum1/2
  Sum1/1 -> Mux/2
  " "/1 -> Product/2
  Gain2/1 -> Product/1
  Product/1 -> Sum1/1
  " 1"/1 -> Product1/2
  Gain1/1 -> Product1/1
  Product1/1 -> Sum/1
  " 2"/1 -> Product2/2
  Product2/1 -> Gain/1
  Product3/1 -> Voltage Control/3(Vz)
  PLL & Measurements/5(Freq) -> Virtual L/1
  Sum2/1 -> Product3/2
  Virtual R/1 -> Sum2/2
  Virtual L/1 -> Sum2/1
  Constant1/1 -> Product2/1

== system MGTestSystem_4bus/Grid-Connected Battery (EMT with Simple Controls)/Battery Controller ==
  m : Inport
  PQref : Inport  Port=2
  Compute PQ : Subsystem
  "P,Q Control " : Subsystem  TreatAsAtomicUnit=on
  to PU : Gain  Gain=1/Pnom
  Idq_ref : Outport  VectorParamsAs1DForOutWhenUnconnected=off
  wires:
  Compute PQ/1(PQm) -> "P,Q Control "/2(m)
  PQref/1 -> to PU/1
  m/1 -> Compute PQ/1(m)
  to PU/1 -> "P,Q Control "/1(PQref)
  "P,Q Control "/1(Idq_ref) -> Idq_ref/1

== system MGTestSystem_4bus/Grid-Connected Battery (EMT with Simple Controls)/DC Link ==
  C1 : spsSeriesRLCBranchLib/Series RLC Branch  LConnTagsString=__new0  RConnTagsString=__new0  BranchType=C  Resistance=1.0  Inductance=1.0  SetiL0=off  InitialCurrent=0  Capacitance=Clink  Setx0=on  InitialVoltage=Vnom_dc/2  Measurements=None
  C2 : spsSeriesRLCBranchLib/Series RLC Branch  LConnTagsString=__new0  RConnTagsString=__new0  BranchType=C  Resistance=1e5  Inductance=1.0  SetiL0=off  InitialCurrent=0  Capacitance=Clink  Setx0=on  InitialVoltage=Vnom_dc/2  Measurements=None
  PV+ : PMIOPort  Side=Left
  PV-- : PMIOPort  Port=2  Side=Left
  Inv+ : PMIOPort  Port=3  Side=Right
  N : PMIOPort  Port=4  Side=Right
  Inv-- : PMIOPort  Port=5  Side=Right
  connections:
  C1/LConn1 -- PV+/RConn1 -- Inv+/RConn1
  C2/LConn1 -- N/RConn1 -- C1/RConn1
  C2/RConn1 -- PV--/RConn1 -- Inv--/RConn1

== system MGTestSystem_4bus/Grid-Connected Battery (EMT with Simple Controls)/Grid Inverter ==
  note: Harmonic Filter
  Uref : Inport
  10 kvar : spsThreePhaseSeriesRLCLoadLib/Three-Phase Series RLC Load  LConnTagsString=A|B|C  Configuration=Delta  NominalVoltage=Vnom_sec  Vabc=[1e3 1e3 1e3]  Vabcp=[1e3 1e3 1e3]  NominalFrequency=Fnom  UnbalancedPower=off  ActivePower=Pc  InductivePower=0  CapacitivePower=Qc  Pabc=[10e3 9e3 11e3]  QLabc=[100 90 110]  QCabc=[100 90 110]  Pabcp=[10e3 9e3 11e3]  QLabcp=[100 90 110]  QCabcp=[100 90 110]  Measurements=None  LoadType=constant Z
  100 kVA 260V / 25 kV : spsThreePhaseTransformerTwoWindingsLib/Three-Phase Transformer (Two Windings)  Winding1Connection=Yg  Winding2Connection=Delta (D1)  CoreType=Three single-phase transformers  SetSaturation=off  Hysteresis=off  DataFile='hysteresis'  SetInitialFlux=off  Measurements=None  UNITS=pu  NominalPower=[Pnom Fnom ]  Winding1=[ Vnom_prim , Rxf/2 , Lxf/2 ]  Winding2=[ Vnom_sec , Rxf/2 , Lxf/2 ]  Rm=200  Lm=200  L0=0.5  Saturation=[ 0,0 ; 0.0024,1.2 ; 1.0,1.52 ]  InitialFluxes=[ 0.8 , -0.8 , 0.7 ]  BreakLoop=off  DiscreteSolver=Trapezoidal iterative  DataType=off  TransfoNumber=0
  B1 : spsThreePhaseVIMeasurementLib/Three-Phase V-I Measurement  VoltageMeasurement=phase-to-ground  SetLabelV=off  LabelV=Vabc_B1  Vpu=off  VpuLL=off  CurrentMeasurement=yes  SetLabelI=off  LabelI=Iabc_B1  Ipu=off  Pbase=100e6  Vbase=500e3  OutputType=Magnitude  PhasorSimulation=off  PSBequivalent=0
  Bus Creator : BusCreator  Inputs=2
  Ground : Ground
  L : spsThreePhaseSeriesRLCBranchLib/Three-Phase Series RLC Branch  LConnTagsString=A|B|C  RConnTagsString=A|B|C  BranchType=RL  Resistance=Rchoke*Zbase  Inductance=Lchoke*Zbase/(2*pi*Fnom)  Capacitance=inf  Measurements=None
  Three-Level NPC Converter : spsThreeLevelNPCConverterLib/Three-Level NPC Converter  ModelType=Average model (Uref-controlled)  Ron=1e-3  Rs=1e6  Cs=inf  Vforward=[0,0]  Ron_Diode=1e-3  Rs_Diode=1e6  Cs_Diode=inf  Vf_Diode=1e-3  Rs_CurrentSource=inf
      settings: SourceProductBaseCode=PS
  Inv+ : PMIOPort  Side=Left
  N : PMIOPort  Port=2  Side=Left
  Inv-- : PMIOPort  Port=3  Side=Left
  A : PMIOPort  Port=4  Side=Right
  B : PMIOPort  Port=5  Side=Right
  C : PMIOPort  Port=6  Side=Right
  m : Outport  VectorParamsAs1DForOutWhenUnconnected=off
  wires:
  Ground/1 -> Three-Level NPC Converter/2
  Bus Creator/1 -> m/1
  B1/2 -> Bus Creator/2  "Iabc"
  B1/1 -> Bus Creator/1  "Vabc"
  Uref/1 -> Three-Level NPC Converter/1
  connections:
  N/RConn1 -- Three-Level NPC Converter/RConn2
  Three-Level NPC Converter/LConn3 -- L/LConn3
  Three-Level NPC Converter/LConn2 -- L/LConn2
  Three-Level NPC Converter/LConn1 -- L/LConn1
  100 kVA 260V / 25 kV/LConn1 -- B1/LConn1
  100 kVA 260V / 25 kV/LConn2 -- B1/LConn2
  100 kVA 260V / 25 kV/LConn3 -- B1/LConn3
  10 kvar/LConn2 -- 100 kVA 260V / 25 kV/RConn2 -- L/RConn2
  10 kvar/LConn3 -- 100 kVA 260V / 25 kV/RConn3 -- L/RConn3
  Three-Level NPC Converter/RConn3 -- Inv--/RConn1
  Three-Level NPC Converter/RConn1 -- Inv+/RConn1
  L/RConn1 -- 100 kVA 260V / 25 kV/RConn1 -- 10 kvar/LConn1
  B1/RConn1 -- A/RConn1
  B1/RConn2 -- B/RConn1
  B1/RConn3 -- C/RConn1

== system MGTestSystem_4bus/Grid-Connected Battery (EMT with Simple Controls)/Inverter Control ==
  Vabc_prim : Inport  PortDimensions=3
  Iabc_prim : Inport  Port=2  PortDimensions=3
  Idq_ref : Inport  Port=3
  Current Control : Subsystem  TreatAsAtomicUnit=on
  Overmodulation : spsOvermodulationLib/Overmodulation  OverModType=Flat top
      settings: SourceProductBaseCode=PS
  PLL & Measurements : Subsystem
  Unit Delay : UnitDelay  SampleTime=Ts_Control  HasFrameUpgradeWarning=on
  Uref : Outport  VectorParamsAs1DForOutWhenUnconnected=off
  wires:
  Vabc_prim/1 -> PLL & Measurements/1(Vabc_prim)
  Iabc_prim/1 -> PLL & Measurements/2(Iabc_prim)
  PLL & Measurements/3(IdIq_prim) -> Current Control/3(IdIq_meas)
  PLL & Measurements/2(VdVq_prim) -> Current Control/2(VdVq_meas)
  PLL & Measurements/1(wt) -> Current Control/1(wt)
  Idq_ref/1 -> Current Control/4(IdIq_ref)
  Current Control/1(Uabc) -> Unit Delay/1
  Overmodulation/1 -> Uref/1
  Unit Delay/1 -> Overmodulation/1

== system MGTestSystem_4bus/Grid-Connected Battery (EMT with Simple Controls)/Measures ==
  Grid : Inport
  Battery : Inport  Port=2
  Bus Creator : BusCreator  Inputs=2
  Bus Creator1 : BusCreator  Inputs=4
  Bus Selector2 : BusSelector  OutputSignals=Vabc,Iabc
  "Power (3ph, Instantaneous)" : spsPower3phInstantaneousLib/Power (3ph, Instantaneous)
  m : Outport  VectorParamsAs1DForOutWhenUnconnected=off
  wires:
  Bus Selector2/1 -> "Power (3ph, Instantaneous)"/1, Bus Creator1/1  "<Vabc>"
  Bus Selector2/2 -> "Power (3ph, Instantaneous)"/2, Bus Creator1/2  "<Iabc>"
  "Power (3ph, Instantaneous)"/1 -> Bus Creator1/3  "P"
  Bus Creator/1 -> m/1
  Battery/1 -> Bus Creator/2  "Battery"
  Grid/1 -> Bus Selector2/1
  "Power (3ph, Instantaneous)"/2 -> Bus Creator1/4  "Q"
  Bus Creator1/1 -> Bus Creator/1  "Grid"

== system MGTestSystem_4bus/Grid-Connected Battery (EMT with Simple Controls)1/Battery Controller ==
  m : Inport
  PQref : Inport  Port=2
  Compute PQ : Subsystem
  "P,Q Control " : Subsystem  TreatAsAtomicUnit=on
  to PU : Gain  Gain=1/Pnom
  Idq_ref : Outport  VectorParamsAs1DForOutWhenUnconnected=off
  wires:
  Compute PQ/1(PQm) -> "P,Q Control "/2(m)
  PQref/1 -> to PU/1
  m/1 -> Compute PQ/1(m)
  to PU/1 -> "P,Q Control "/1(PQref)
  "P,Q Control "/1(Idq_ref) -> Idq_ref/1
